simulink model "JKFF_MS"  (R2025a)
settings: Solver=VariableStepAuto  StartTime=0.0  StopTime=Inf  RelTol=1e-3
libraries: simulink_extras x1
settings Model: Creator=Soochan Kim  LastModifiedBy=Soochan Kim

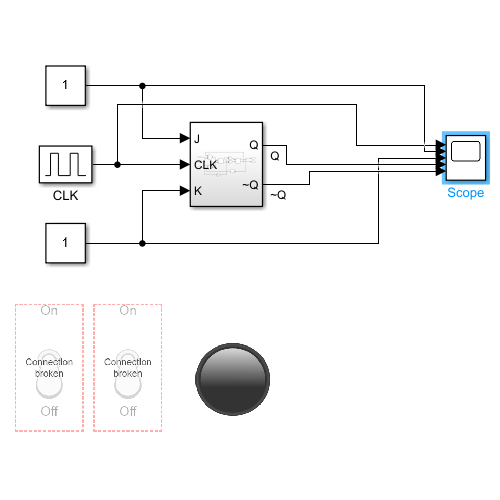
[thumbnail: Simulink's stored preview of the top-level diagram]
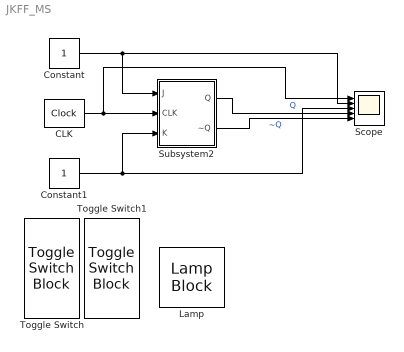
== system JKFF_MS ==
  CLK : simulink_extras/Flip Flops/Clock  period=0.5
  Constant : Constant
  Constant1 : Constant
  Lamp : LampBlock  LabelPosition=Hide  DefaultColor=[192.0, 192.0, 192.0]
  Scope : Scope  NumInputPorts=5
      settings: ActiveDisplayYMinimum=-0.12499999999999997  ActiveDisplayYMaximum=1.125
  Subsystem2 : Subsystem
  Toggle Switch : ToggleSwitchBlock
  Toggle Switch1 : ToggleSwitchBlock
  wires:
  CLK/1 -> Scope/1, Subsystem2/2(CLK)
  Subsystem2/1(Q) -> Scope/4  "Q"
  Constant/1 -> Scope/2, Subsystem2/1(J)
  Constant1/1 -> Subsystem2/3(K), Scope/3
  Subsystem2/2(~Q) -> Scope/5  "~Q"

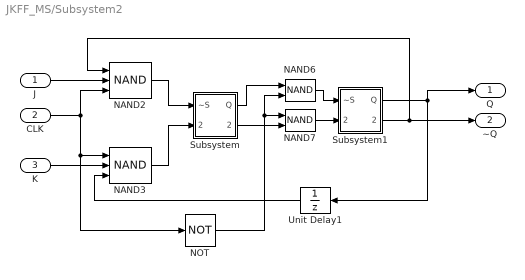
== system JKFF_MS/Subsystem2 ==
  J : Inport
  CLK : Inport  Port=2
  K : Inport  Port=3
  NAND2 : Logic  Operator=NAND  Inputs=3  IconShape=distinctive  AllPortsSameDT=off  OutDataTypeStr=boolean
  NAND3 : Logic  Operator=NAND  Inputs=3  IconShape=distinctive  AllPortsSameDT=off  OutDataTypeStr=boolean
  NAND6 : Logic  Operator=NAND  IconShape=distinctive  AllPortsSameDT=off  OutDataTypeStr=boolean
  NAND7 : Logic  Operator=NAND  IconShape=distinctive  AllPortsSameDT=off  OutDataTypeStr=boolean
  NOT : Logic  Operator=NOT  IconShape=distinctive  AllPortsSameDT=off  OutDataTypeStr=boolean
  Subsystem : Subsystem
  Subsystem1 : Subsystem
  Unit Delay1 : UnitDelay  SampleTime=-1  HasFrameUpgradeWarning=on
  Q : Outport
  ~Q : Outport  Port=2
  wires:
  CLK/1 -> NAND2/3, NAND3/1, NOT/1
  K/1 -> NAND3/2
  J/1 -> NAND2/2
  Unit Delay1/1 -> NAND3/3
  NOT/1 -> NAND7/1, NAND6/2
  NAND2/1 -> Subsystem/1(~S)
  NAND3/1 -> Subsystem/2(~R)
  Subsystem/1(Q) -> NAND6/1
  Subsystem/2(~Q) -> NAND7/2
  NAND6/1 -> Subsystem1/1(~S)
  NAND7/1 -> Subsystem1/2(~R)
  Subsystem1/2(~Q) -> NAND2/1, ~Q/1
  Subsystem1/1(Q) -> Unit Delay1/1, Q/1

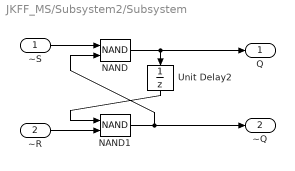
== system JKFF_MS/Subsystem2/Subsystem ==
  ~S : Inport
  ~R : Inport  Port=2
  NAND : Logic  Operator=NAND  IconShape=distinctive  AllPortsSameDT=off  OutDataTypeStr=boolean
  NAND1 : Logic  Operator=NAND  IconShape=distinctive  AllPortsSameDT=off  OutDataTypeStr=boolean
  Unit Delay2 : UnitDelay  SampleTime=-1  HasFrameUpgradeWarning=on
  Q : Outport
  ~Q : Outport  Port=2
  wires:
  NAND/1 -> Q/1, Unit Delay2/1
  NAND1/1 -> ~Q/1, NAND/2
  Unit Delay2/1 -> NAND1/1
  ~S/1 -> NAND/1
  ~R/1 -> NAND1/2

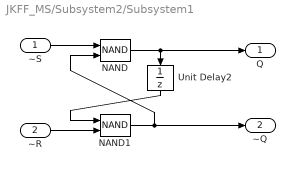
== system JKFF_MS/Subsystem2/Subsystem1 ==
  ~S : Inport
  ~R : Inport  Port=2
  NAND : Logic  Operator=NAND  IconShape=distinctive  AllPortsSameDT=off  OutDataTypeStr=boolean
  NAND1 : Logic  Operator=NAND  IconShape=distinctive  AllPortsSameDT=off  OutDataTypeStr=boolean
  Unit Delay2 : UnitDelay  SampleTime=-1  HasFrameUpgradeWarning=on
  Q : Outport
  ~Q : Outport  Port=2
  wires:
  NAND/1 -> Q/1, Unit Delay2/1
  NAND1/1 -> ~Q/1, NAND/2
  Unit Delay2/1 -> NAND1/1
  ~S/1 -> NAND/1
  ~R/1 -> NAND1/2
